simulink model "simulation_fuzzy_final_G4"  (R2020a)
settings: Solver=VariableStepAuto  StartTime=0.0  StopTime=150  RelTol=1e-3
libraries: fuzblock x1
settings Model: Creator=Ayush Agrawal  LastModifiedBy=Ayush Agrawal
settings SolverCC: ZeroCrossAlgorithm=Adaptive
settings DebuggingCC: MaskedZcDiagnostic=none  IgnoredZcDiagnostic=none

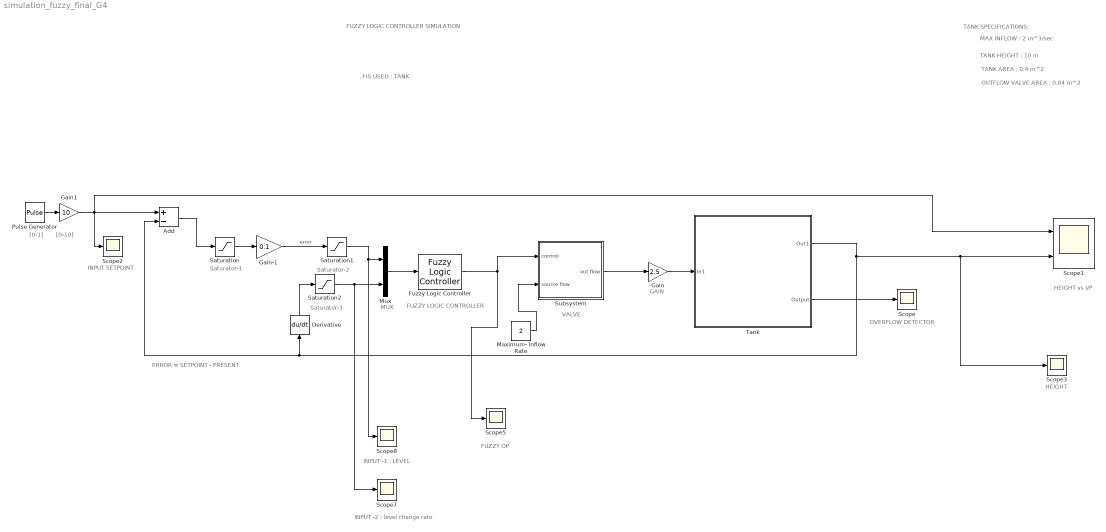
== system simulation_fuzzy_final_G4 ==
  note: . FIS USED : TANK
  note: FUZZY LOGIC CONTROLLER SIMULATION
  note: Saturator-3
  note: Saturator-2
  note: Saturator-1
  note: TANK SPECIFICATIONS:
  note: GAIN
  note: HEIGHT
  note: ERROR = SETPOINT - PRESENT
  note: [0-1]
  note: FUZZY OP
  note: TANK AREA : 0.4 m^2
  note: MAX INFLOW : 2 m^3/sec
  note: INPUT -1 : LEVEL
  note: OVERFLOW DETECTOR
  note: OUTFLOW VALVE AREA : 0.04 m^2
  note: INPUT SETPOINT
  note: HEIGHT vs I/P
  note: VALVE
  note: INPUT -2 : level change rate
  note: [0-10]
  note: MUX
  note: FUZZY LOGIC CONTROLLER
  note: TANK HEIGHT : 10 m
  "Add " : Sum  Inputs=+-
  Derivative : Derivative
  Fuzzy Logic Controller : fuzblock/Fuzzy Logic  Controller  FIS=tank  OutputSampleNumber=101  DataType=double  FuzzifiedInputs=off  RuleFiringStrengths=off  RuleOutputs=off  AggregatedOutputs=off  SimulateUsing=Interpreted execution  OutOfRangeInputValueMessage=warning  NoRuleFiredMessage=warning  EmptyOutputFuzzySetMessage=warning
  Gain : Gain  Gain=2.5
  Gain-1 : Gain  Gain=0.1
  Gain1 : Gain  Gain=10
  Maximum- Inflow Rate : Constant  Value=2
  Mux : Mux  Inputs=2
  Pulse Generator : DiscretePulseGenerator  PulseType=Time based  Period=100  PulseWidth=50
  Saturation : Saturate  UpperLimit=10  LowerLimit=-10  OutMin=-10  OutMax=10
  Saturation1 : Saturate  UpperLimit=1.1  LowerLimit=-1.1  LinearizeAsGain=off  ZeroCross=off  OutMin=-1.1  OutMax=1.1
  Saturation2 : Saturate  UpperLimit=0.35  LowerLimit=-0.35  ZeroCross=off  OutMin=-0.35  OutMax=0.35
  Scope{,2..3,5,7..8} (6 alike) : Scope
  Scope1 : Scope  NumInputPorts=2
  Subsystem : Subsystem  mask(Valve){InitialPosition=0}
      mask prompts: InitialPosition "Initial position [0=closed 1=open]:"
      mask help: Valve
      mask Display: image('$imagefile'); % Use "Edit Image" on toolstrip to change.
  Tank : Subsystem  mask{ht=10, Tarea=0.4, Oarea=0.04, initialHt=0.0, overflowLimit=0}
      mask prompts: ht "Height of Tank(m)"; Tarea "Tank Area (m^2)"; Oarea "Outflow Cross-Section Area(m^2)"; initialHt "Initial Level Height(m)"; overflowLimit "Overflow Sensor distance from top(m)"
      mask Display: image('$imagefile'); % Use "Edit Image" on toolstrip to change.
  wires:
  Tank/2(Output) -> Scope/1
  Saturation/1 -> Gain-1/1
  Derivative/1 -> Saturation2/1
  Saturation2/1 -> Scope7/1, Mux/2
  Saturation1/1 -> Scope8/1, Mux/1
  Gain1/1 -> "Add "/1, Scope1/1, Scope2/1
  Gain/1 -> Tank/1(In1)
  Tank/1(Out1) -> Derivative/1, "Add "/2, Scope3/1, Scope1/2
  Fuzzy Logic Controller/1 -> Scope5/1, Subsystem/1(control)
  Pulse Generator/1 -> Gain1/1
  "Add "/1 -> Saturation/1
  Mux/1 -> Fuzzy Logic Controller/1
  Gain-1/1 -> Saturation1/1  "error"
  Maximum- Inflow Rate/1 -> Subsystem/2(source flow)
  Subsystem/1(out flow) -> Gain/1

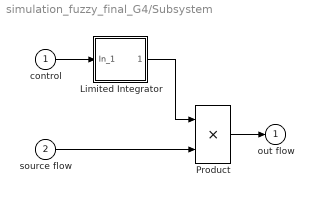
== system simulation_fuzzy_final_G4/Subsystem ==
  control : Inport
  source flow : Inport  Port=2
  Limited Integrator : Subsystem  mask(Limited integrator.){lb=0, ub=1, xi=InitialPosition}
      mask prompts: lb "Lower bound:"; ub "Upper bound:"; xi "Initial condition"
      mask help: Limited integrator
      mask Help: Implements a limited integrator with \nan expression of the form:\n\nif(x<=lb and u<0) or (x>=ub and u>0)\n\txdot=0\nelse\n\txdot=u.
      mask Display: plot(-1,-0.2,3.5,1.2,[0.05,1,2,2.9],[0,0,1,1]);disp(' 1/s    ')
  Product : Product  InputSameDT=on  RndMeth=Zero  SaturateOnIntegerOverflow=on  OutDataTypeStr=Inherit: Same as first input
  out flow : Outport  InitialOutput=0  VectorParamsAs1DForOutWhenUnconnected=off
  wires:
  source flow/1 -> Product/2
  Product/1 -> out flow/1
  control/1 -> Limited Integrator/1(In_1)
  Limited Integrator/1(Out_1) -> Product/1

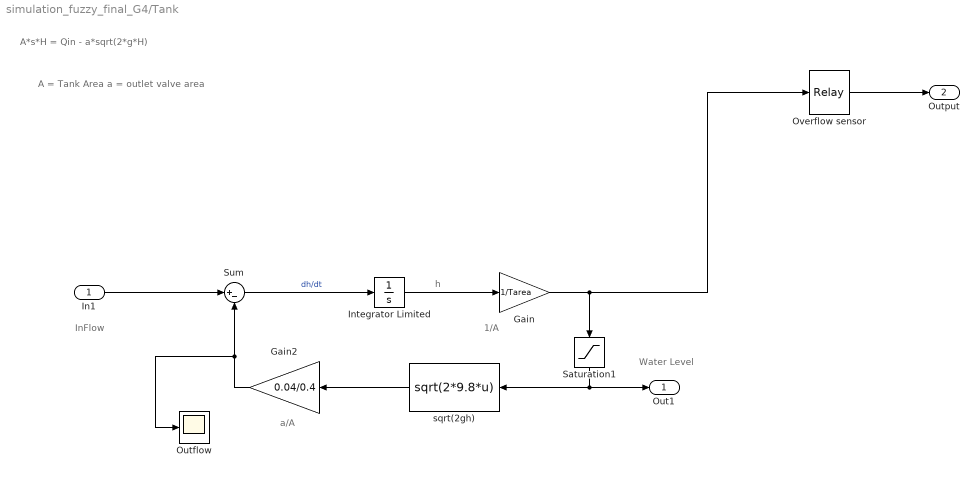
== system simulation_fuzzy_final_G4/Tank ==
  note: 1/A
  note: A = Tank Area
      | a = outlet valve area
  note: h
  note: A*s*H = Qin - a*sqrt(2*g*H)
  note: a/A
  note: InFlow
  note: Water Level
  In1 : Inport
  Gain : Gain  Gain=1/Tarea
  Gain2 : Gain  Gain=0.04/0.4
  Integrator Limited : Integrator  LimitOutput=on  UpperSaturationLimit=ht*Tarea  LowerSaturationLimit=0
  Outflow : Scope
  Overflow sensor : Relay  OnSwitchValue=ht - overflowLimit  OffSwitchValue=0  OnOutputValue=0  OffOutputValue=1
  Saturation1 : Saturate  UpperLimit=10  LowerLimit=0  OutMin=0  OutMax=10
  Sum : Sum  Inputs=|+-
  sqrt(2gh) : Fcn  Expr=sqrt(2*9.8*u)
  Out1 : Outport
  Output : Outport  Port=2
  wires:
  Overflow sensor/1 -> Output/1
  In1/1 -> Sum/1
  Gain2/1 -> Outflow/1, Sum/2
  Gain/1 -> Overflow sensor/1, Saturation1/1
  Sum/1 -> Integrator Limited/1  "dh/dt"
  Integrator Limited/1 -> Gain/1
  Saturation1/1 -> sqrt(2gh)/1, Out1/1
  sqrt(2gh)/1 -> Gain2/1

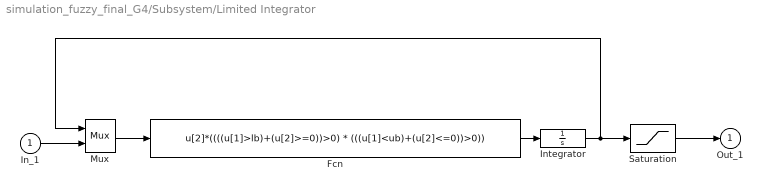
== system simulation_fuzzy_final_G4/Subsystem/Limited Integrator ==
  In_1 : Inport
  Fcn : Fcn  Expr=u[2]*((((u[1]>lb)+(u[2]>=0))>0) * (((u[1]<ub)+(u[2]<=0))>0))
  Integrator : Integrator  InitialCondition=xi
  Mux : Mux  Inputs=2
  Saturation : Saturate  UpperLimit=ub  LowerLimit=lb
  Out_1 : Outport  InitialOutput=0  VectorParamsAs1DForOutWhenUnconnected=off
  wires:
  Integrator/1 -> Saturation/1, Mux/1
  Fcn/1 -> Integrator/1
  Mux/1 -> Fcn/1
  In_1/1 -> Mux/2
  Saturation/1 -> Out_1/1
